simulink model "psbsixpulses"  (Simulink 6.0)
settings: Solver=ode23s  SolverMode=SingleTasking  StartTime=0.0  StopTime=0.035  RelTol=1e-5  AbsTol=1e-5
InitFcn:
  | powericon('psbinitsys',bdroot);
libraries: powerlib2 x14, powerlib_extras x1
settings Model: Creator=sybille  LastModifiedBy=batserve  ExtModeTrigMode=oneshot  ExtModeArmWhenConnect=off  ExtModeAutoUpdateStatusClock=off
settings SolverCC: MaxOrder=1
settings DataIOCC: LimitDataPoints=off  SaveOutput=off  SaveTime=off  SignalLoggingName=sigsOut
settings OptimizationCC: BlockReduction=off  BooleanDataType=off
settings DebuggingCC: SolverPrmCheckMsg=none  UnconnectedInputMsg=none  UnconnectedOutputMsg=none
settings HardwareCC: TargetUnknown=on
settings RTWCC: TemplateMakefile=grt_unix.tmf

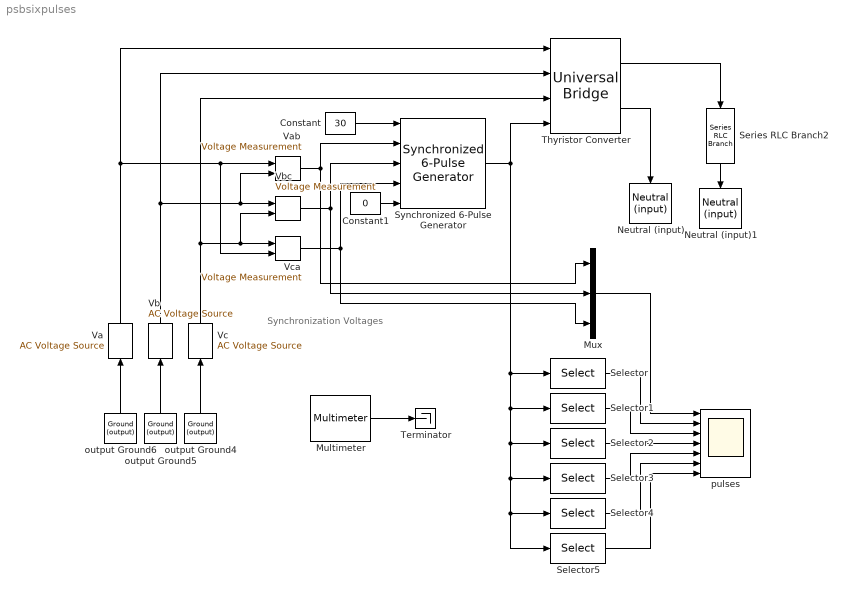
== system psbsixpulses ==
  note: Synchronization Voltages
  Constant : Constant  Value=30
  Constant1 : Constant  Value=0
  Multimeter : powerlib2/Measurements/Multimeter  Tag=PoWeRsYsTeMmEaSuReMeNt  PhasorSimulation=off  OutputType=Magnitude  sel=[1 2 3 4 5 6 9]  L=15  Gain=[-1 -1 -1 -1 -1 -1 1]  yselected={'Usw1: Thyristor Converter','Usw2: Thyristor Converter','Usw3: Thyristor Converter','Usw4: Thyristor Converter','Usw5: Thyristor Converter','Usw6: Thyristor Converter','Udc: Thyristor Converter'};  PSBOutputType=1  PSBequivalent=0  AxesSetting=[0,0.1,-100,100]  Display=1  SavedBlockNames=-11
  Mux : Mux  Inputs=3
  Neutral (input) : powerlib2/Connectors/Neutral (input)  Tag=PoWeRsYsTeMbLoCk  Orientation=down  no=1
  Neutral (input)1 : powerlib2/Connectors/Neutral (input)  Tag=PoWeRsYsTeMbLoCk  Orientation=down  no=1
  Selector : Selector  InputPortWidth=6
  Selector1 : Selector  Elements=2  InputPortWidth=6
  Selector2 : Selector  Elements=3  InputPortWidth=6
  Selector3 : Selector  Elements=4  InputPortWidth=6
  Selector4 : Selector  Elements=5  InputPortWidth=6
  Selector5 : Selector  Elements=6  InputPortWidth=6
  Series RLC Branch2 : powerlib2/Elements/Series RLC Branch  Tag=PoWeRsYsTeMbLoCk  Orientation=down  a=2  b=0  c=inf  mesure=None  PSBOutputType=1
  Synchronized 6-Pulse Generator : powerlib_extras/Control  Blocks/Synchronized 6-Pulse Generator  freq=60  pwidth=10  Double_Pulse=on
  Terminator : Terminator
  Thyristor Converter : powerlib2/Power Electronics/Universal Bridge  Tag=PoWeRsYsTeMbLoCk  arms=3  confi=ABC as input terminals  injcc=500  cf=1e-6  device=Thyristors  Ron=1e-3  Lon=0  VFs="[  0.8  0.8  ]"  Vf=0  gtoparameters=[ 10e-6 , 20e-6 ]  igbtparameters=[ 1e-6 , 2e-6 ]  mesure=All voltages and currents  PSBOutputType=111
  Va : powerlib2/Electrical Sources/AC Voltage Source  Tag=PoWeRsYsTeMbLoCk  Orientation=up  A=200  P=0  F=60  stime=0  mesure=None  PSBOutputType=1
  Vab : powerlib2/Measurements/Voltage Measurement  Tag=PoWeRsYsTeMmEaSuReMeNt  PhasorSimulation=off  OutputType=Magnitude  PSBOutputType=0  PSBequivalent=0
  Vb : powerlib2/Electrical Sources/AC Voltage Source  Tag=PoWeRsYsTeMbLoCk  Orientation=up  A=200  P=-120  F=60  stime=0  mesure=None  PSBOutputType=1
  Vbc : powerlib2/Measurements/Voltage Measurement  Tag=PoWeRsYsTeMmEaSuReMeNt  PhasorSimulation=off  OutputType=Magnitude  PSBOutputType=0  PSBequivalent=0
  Vc : powerlib2/Electrical Sources/AC Voltage Source  Tag=PoWeRsYsTeMbLoCk  Orientation=up  A=200  P=120  F=60  stime=0  mesure=None  PSBOutputType=1
  Vca : powerlib2/Measurements/Voltage Measurement  Tag=PoWeRsYsTeMmEaSuReMeNt  PhasorSimulation=off  OutputType=Magnitude  PSBOutputType=0  PSBequivalent=0
  output Ground4 : powerlib2/Connectors/Ground (output)  Tag=PoWeRsYsTeMbLoCk  Orientation=up  PSBOutputType=1
  output Ground5 : powerlib2/Connectors/Ground (output)  Tag=PoWeRsYsTeMbLoCk  Orientation=up  PSBOutputType=1
  output Ground6 : powerlib2/Connectors/Ground (output)  Tag=PoWeRsYsTeMbLoCk  Orientation=up  PSBOutputType=1
  pulses : Scope  NumInputPorts=7
      settings: TimeRange=0.035  YMin=-400~-1~-1~-1~0~0~0  YMax=400~1~1~1~1~1~1  SaveName=VI_scope  SampleInput=on  SampleTime=1/60/512
  wires:
  Thyristor Converter/1 -> Series RLC Branch2/1
  output Ground6/1 -> Va/1
  output Ground5/1 -> Vb/1
  output Ground4/1 -> Vc/1
  Thyristor Converter/2 -> Neutral (input)/1
  Series RLC Branch2/1 -> Neutral (input)1/1
  Vb/1 -> Vbc/1, Vab/2, Thyristor Converter/2
  Vc/1 -> Vca/1, Vbc/2, Thyristor Converter/3
  Va/1 -> Vab/1, Vca/2, Thyristor Converter/1
  Vca/1 -> Synchronized 6-Pulse Generator/4, Mux/3
  Vbc/1 -> Synchronized 6-Pulse Generator/3, Mux/2
  Vab/1 -> Synchronized 6-Pulse Generator/2, Mux/1
  Constant/1 -> Synchronized 6-Pulse Generator/1
  Synchronized 6-Pulse Generator/1 -> Thyristor Converter/4, Selector/1, Selector1/1, Selector2/1, Selector3/1, Selector5/1, Selector4/1
  Selector5/1 -> pulses/7
  Selector4/1 -> pulses/6
  Selector3/1 -> pulses/5
  Selector2/1 -> pulses/4
  Selector1/1 -> pulses/3
  Selector/1 -> pulses/2
  Mux/1 -> pulses/1
  Constant1/1 -> Synchronized 6-Pulse Generator/5
  Multimeter/1 -> Terminator/1
